simulink model "PID_SingleJoint"  (R2018b)
settings: Solver=FixedStepDiscrete  StartTime=0.0  StopTime=Inf  FixedStep=0.001  RelTol=1e-3  EnableMultiTasking=on
undefined symbols (not defined in the file): DiscIntNeverNeededParam, J1, J2, J3, J4, J5, J6, J7, Motor_Current, Motor_Position, Motor_Velocity, q, qd, Send_GUIdata, Tau
libraries: c280xlib x14, simulink x11, dspsrcs4 x6, idelinklib_common x1
(part 3 of 4)

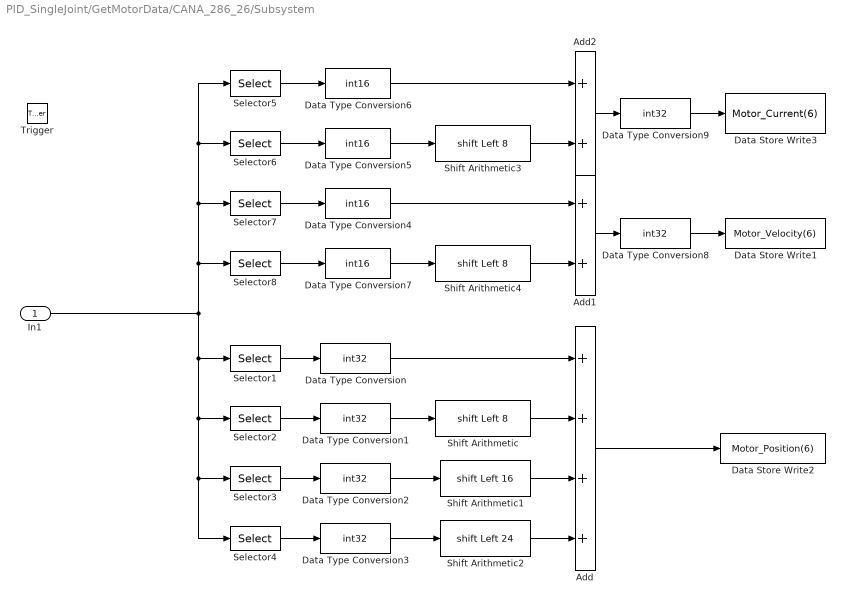
== system PID_SingleJoint/GetMotorData/CANA_286_26/Subsystem ==
  In1 : Inport
  Trigger : TriggerPort  TriggerType=function-call  VariantControl=Variant  PortDimensions=1
  Add : Sum  Inputs=4
  Add1 : Sum  Inputs=2
  Add2 : Sum  Inputs=2
  Data Store Write1 : DataStoreWrite  DataStoreName=Motor_Velocity  DataStoreElements=Motor_Velocity(6)
  Data Store Write2 : DataStoreWrite  DataStoreName=Motor_Position  DataStoreElements=Motor_Position(6)
  Data Store Write3 : DataStoreWrite  DataStoreName=Motor_Current  DataStoreElements=Motor_Current(6)
  Data Type Conversion{,1..3,8..9} (6 alike) : DataTypeConversion  OutDataTypeStr=int32
  Data Type Conversion{4..7} (4 alike) : DataTypeConversion  OutDataTypeStr=int16
  Selector1 : Selector  IndexMode=Zero-based  InputPortWidth=8  IndexOptions=Index vector (dialog)  Indices=4  OutputSizes=1
  Selector2 : Selector  IndexMode=Zero-based  InputPortWidth=8  IndexOptions=Index vector (dialog)  Indices=5  OutputSizes=1
  Selector3 : Selector  IndexMode=Zero-based  InputPortWidth=8  IndexOptions=Index vector (dialog)  Indices=6  OutputSizes=1
  Selector4 : Selector  IndexMode=Zero-based  InputPortWidth=8  IndexOptions=Index vector (dialog)  Indices=7  OutputSizes=1
  Selector5 : Selector  IndexMode=Zero-based  InputPortWidth=8  IndexOptions=Index vector (dialog)  Indices=0  OutputSizes=1
  Selector6 : Selector  IndexMode=Zero-based  InputPortWidth=8  IndexOptions=Index vector (dialog)  Indices=1  OutputSizes=1
  Selector7 : Selector  IndexMode=Zero-based  InputPortWidth=8  IndexOptions=Index vector (dialog)  Indices=2  OutputSizes=1
  Selector8 : Selector  IndexMode=Zero-based  InputPortWidth=8  IndexOptions=Index vector (dialog)  Indices=3  OutputSizes=1
  Shift Arithmetic : ArithShift  BitShiftNumber=8  BitShiftDirection=Left
  Shift Arithmetic1 : ArithShift  BitShiftNumber=16  BitShiftDirection=Left
  Shift Arithmetic2 : ArithShift  BitShiftNumber=24  BitShiftDirection=Left
  Shift Arithmetic3 : ArithShift  BitShiftNumber=8  BitShiftDirection=Left
  Shift Arithmetic4 : ArithShift  BitShiftNumber=8  BitShiftDirection=Left
  wires:
  Selector3/1 -> Data Type Conversion2/1
  Shift Arithmetic/1 -> Add/2
  Shift Arithmetic2/1 -> Add/4
  Data Type Conversion/1 -> Add/1
  Selector1/1 -> Data Type Conversion/1
  Selector4/1 -> Data Type Conversion3/1
  Add/1 -> Data Store Write2/1
  Shift Arithmetic1/1 -> Add/3
  Selector2/1 -> Data Type Conversion1/1
  Selector5/1 -> Data Type Conversion6/1
  Data Type Conversion7/1 -> Shift Arithmetic4/1
  Selector7/1 -> Data Type Conversion4/1
  Selector8/1 -> Data Type Conversion7/1
  Selector6/1 -> Data Type Conversion5/1
  In1/1 -> Selector3/1, Selector4/1, Selector2/1, Selector1/1, Selector5/1, Selector6/1, Selector7/1, Selector8/1
  Add1/1 -> Data Type Conversion8/1
  Data Type Conversion1/1 -> Shift Arithmetic/1
  Data Type Conversion2/1 -> Shift Arithmetic1/1
  Data Type Conversion3/1 -> Shift Arithmetic2/1
  Shift Arithmetic4/1 -> Add1/2
  Data Type Conversion4/1 -> Add1/1
  Data Type Conversion5/1 -> Shift Arithmetic3/1
  Data Type Conversion6/1 -> Add2/1
  Shift Arithmetic3/1 -> Add2/2
  Add2/1 -> Data Type Conversion9/1
  Data Type Conversion8/1 -> Data Store Write1/1
  Data Type Conversion9/1 -> Data Store Write3/1

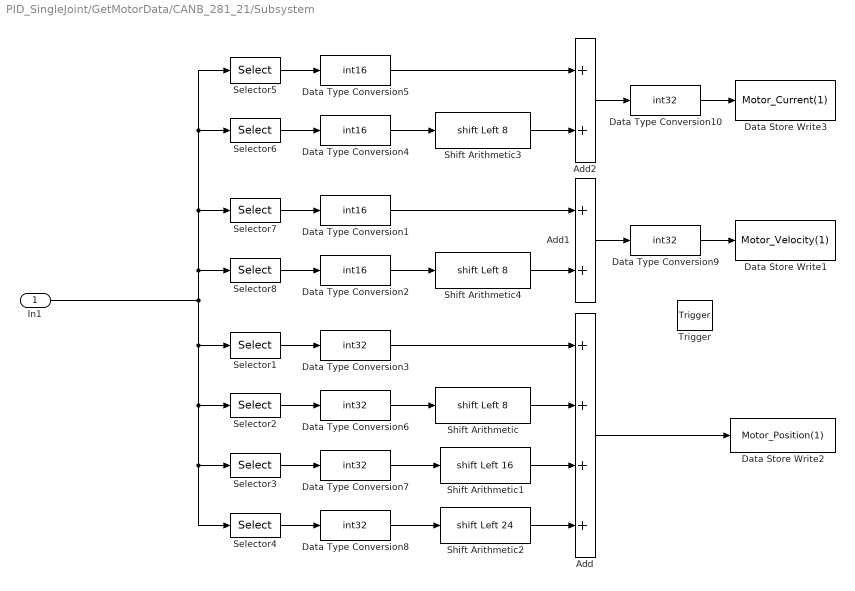
== system PID_SingleJoint/GetMotorData/CANB_281_21/Subsystem ==
  In1 : Inport
  Trigger : TriggerPort  TriggerType=function-call  VariantControl=Variant  PortDimensions=1
  Add : Sum  Inputs=4
  Add1 : Sum  Inputs=2
  Add2 : Sum  Inputs=2
  Data Store Write1 : DataStoreWrite  DataStoreName=Motor_Velocity  DataStoreElements=Motor_Velocity(1)
  Data Store Write2 : DataStoreWrite  DataStoreName=Motor_Position  DataStoreElements=Motor_Position(1)
  Data Store Write3 : DataStoreWrite  DataStoreName=Motor_Current  DataStoreElements=Motor_Current(1)
  Data Type Conversion{1..2,4..5} (4 alike) : DataTypeConversion  OutDataTypeStr=int16
  Data Type Conversion{3,6..10} (6 alike) : DataTypeConversion  OutDataTypeStr=int32
  Selector1 : Selector  IndexMode=Zero-based  InputPortWidth=8  IndexOptions=Index vector (dialog)  Indices=4  OutputSizes=1
  Selector2 : Selector  IndexMode=Zero-based  InputPortWidth=8  IndexOptions=Index vector (dialog)  Indices=5  OutputSizes=1
  Selector3 : Selector  IndexMode=Zero-based  InputPortWidth=8  IndexOptions=Index vector (dialog)  Indices=6  OutputSizes=1
  Selector4 : Selector  IndexMode=Zero-based  InputPortWidth=8  IndexOptions=Index vector (dialog)  Indices=7  OutputSizes=1
  Selector5 : Selector  IndexMode=Zero-based  InputPortWidth=8  IndexOptions=Index vector (dialog)  Indices=0  OutputSizes=1
  Selector6 : Selector  IndexMode=Zero-based  InputPortWidth=8  IndexOptions=Index vector (dialog)  Indices=1  OutputSizes=1
  Selector7 : Selector  IndexMode=Zero-based  InputPortWidth=8  IndexOptions=Index vector (dialog)  Indices=2  OutputSizes=1
  Selector8 : Selector  IndexMode=Zero-based  InputPortWidth=8  IndexOptions=Index vector (dialog)  Indices=3  OutputSizes=1
  Shift Arithmetic : ArithShift  BitShiftNumber=8  BitShiftDirection=Left
  Shift Arithmetic1 : ArithShift  BitShiftNumber=16  BitShiftDirection=Left
  Shift Arithmetic2 : ArithShift  BitShiftNumber=24  BitShiftDirection=Left
  Shift Arithmetic3 : ArithShift  BitShiftNumber=8  BitShiftDirection=Left
  Shift Arithmetic4 : ArithShift  BitShiftNumber=8  BitShiftDirection=Left
  wires:
  Data Type Conversion7/1 -> Shift Arithmetic1/1
  Shift Arithmetic/1 -> Add/2
  Selector2/1 -> Data Type Conversion6/1
  Selector3/1 -> Data Type Conversion7/1
  Shift Arithmetic2/1 -> Add/4
  Data Type Conversion3/1 -> Add/1
  Selector1/1 -> Data Type Conversion3/1
  Data Type Conversion8/1 -> Shift Arithmetic2/1
  Add/1 -> Data Store Write2/1
  Selector4/1 -> Data Type Conversion8/1
  Shift Arithmetic1/1 -> Add/3
  Data Type Conversion6/1 -> Shift Arithmetic/1
  Data Type Conversion2/1 -> Shift Arithmetic4/1
  Shift Arithmetic4/1 -> Add1/2
  Data Type Conversion1/1 -> Add1/1
  Selector7/1 -> Data Type Conversion1/1
  Selector8/1 -> Data Type Conversion2/1
  Selector6/1 -> Data Type Conversion4/1
  In1/1 -> Selector3/1, Selector4/1, Selector2/1, Selector1/1, Selector5/1, Selector6/1, Selector7/1, Selector8/1
  Add1/1 -> Data Type Conversion9/1
  Selector5/1 -> Data Type Conversion5/1
  Data Type Conversion4/1 -> Shift Arithmetic3/1
  Data Type Conversion9/1 -> Data Store Write1/1
  Shift Arithmetic3/1 -> Add2/2
  Data Type Conversion5/1 -> Add2/1
  Add2/1 -> Data Type Conversion10/1
  Data Type Conversion10/1 -> Data Store Write3/1

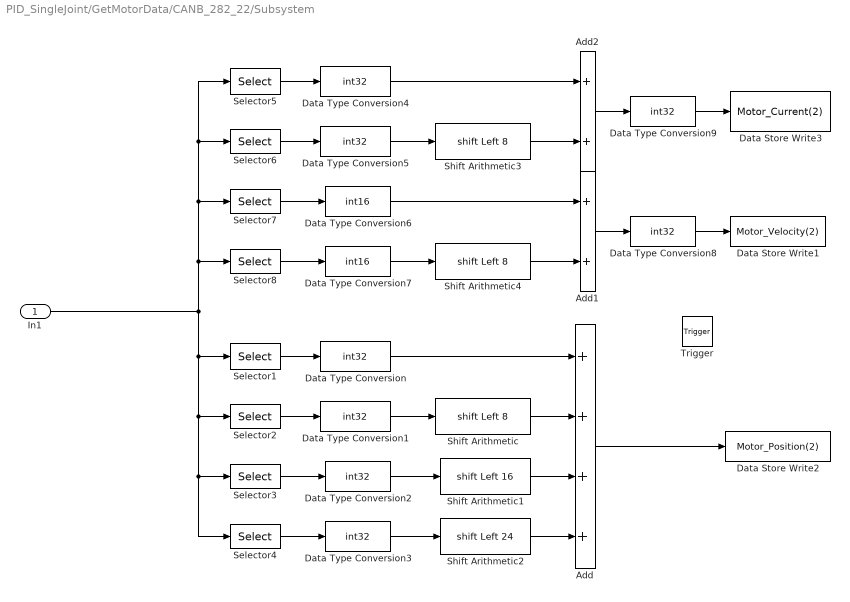
== system PID_SingleJoint/GetMotorData/CANB_282_22/Subsystem ==
  In1 : Inport
  Trigger : TriggerPort  TriggerType=function-call  VariantControl=Variant  PortDimensions=1
  Add : Sum  Inputs=4
  Add1 : Sum  Inputs=2
  Add2 : Sum  Inputs=2
  Data Store Write1 : DataStoreWrite  DataStoreName=Motor_Velocity  DataStoreElements=Motor_Velocity(2)
  Data Store Write2 : DataStoreWrite  DataStoreName=Motor_Position  DataStoreElements=Motor_Position(2)
  Data Store Write3 : DataStoreWrite  DataStoreName=Motor_Current  DataStoreElements=Motor_Current(2)
  Data Type Conversion{,1..5,8..9} (8 alike) : DataTypeConversion  OutDataTypeStr=int32
  Data Type Conversion6 : DataTypeConversion  OutDataTypeStr=int16
  Data Type Conversion7 : DataTypeConversion  OutDataTypeStr=int16
  Selector1 : Selector  IndexMode=Zero-based  InputPortWidth=8  IndexOptions=Index vector (dialog)  Indices=4  OutputSizes=1
  Selector2 : Selector  IndexMode=Zero-based  InputPortWidth=8  IndexOptions=Index vector (dialog)  Indices=5  OutputSizes=1
  Selector3 : Selector  IndexMode=Zero-based  InputPortWidth=8  IndexOptions=Index vector (dialog)  Indices=6  OutputSizes=1
  Selector4 : Selector  IndexMode=Zero-based  InputPortWidth=8  IndexOptions=Index vector (dialog)  Indices=7  OutputSizes=1
  Selector5 : Selector  IndexMode=Zero-based  InputPortWidth=8  IndexOptions=Index vector (dialog)  Indices=0  OutputSizes=1
  Selector6 : Selector  IndexMode=Zero-based  InputPortWidth=8  IndexOptions=Index vector (dialog)  Indices=1  OutputSizes=1
  Selector7 : Selector  IndexMode=Zero-based  InputPortWidth=8  IndexOptions=Index vector (dialog)  Indices=2  OutputSizes=1
  Selector8 : Selector  IndexMode=Zero-based  InputPortWidth=8  IndexOptions=Index vector (dialog)  Indices=3  OutputSizes=1
  Shift Arithmetic : ArithShift  BitShiftNumber=8  BitShiftDirection=Left
  Shift Arithmetic1 : ArithShift  BitShiftNumber=16  BitShiftDirection=Left
  Shift Arithmetic2 : ArithShift  BitShiftNumber=24  BitShiftDirection=Left
  Shift Arithmetic3 : ArithShift  BitShiftNumber=8  BitShiftDirection=Left
  Shift Arithmetic4 : ArithShift  BitShiftNumber=8  BitShiftDirection=Left
  wires:
  Data Type Conversion2/1 -> Shift Arithmetic1/1
  Shift Arithmetic/1 -> Add/2
  Selector2/1 -> Data Type Conversion1/1
  Selector3/1 -> Data Type Conversion2/1
  Shift Arithmetic2/1 -> Add/4
  Data Type Conversion/1 -> Add/1
  Selector1/1 -> Data Type Conversion/1
  Data Type Conversion3/1 -> Shift Arithmetic2/1
  Add/1 -> Data Store Write2/1
  Selector4/1 -> Data Type Conversion3/1
  Shift Arithmetic1/1 -> Add/3
  Data Type Conversion1/1 -> Shift Arithmetic/1
  In1/1 -> Selector3/1, Selector4/1, Selector2/1, Selector1/1, Selector8/1, Selector7/1, Selector6/1, Selector5/1
  Shift Arithmetic4/1 -> Add1/2
  Add1/1 -> Data Type Conversion8/1
  Data Type Conversion5/1 -> Shift Arithmetic3/1
  Selector8/1 -> Data Type Conversion7/1
  Data Type Conversion6/1 -> Add1/1
  Selector6/1 -> Data Type Conversion5/1
  Data Type Conversion7/1 -> Shift Arithmetic4/1
  Selector5/1 -> Data Type Conversion4/1
  Selector7/1 -> Data Type Conversion6/1
  Data Type Conversion8/1 -> Data Store Write1/1
  Shift Arithmetic3/1 -> Add2/2
  Data Type Conversion4/1 -> Add2/1
  Add2/1 -> Data Type Conversion9/1
  Data Type Conversion9/1 -> Data Store Write3/1

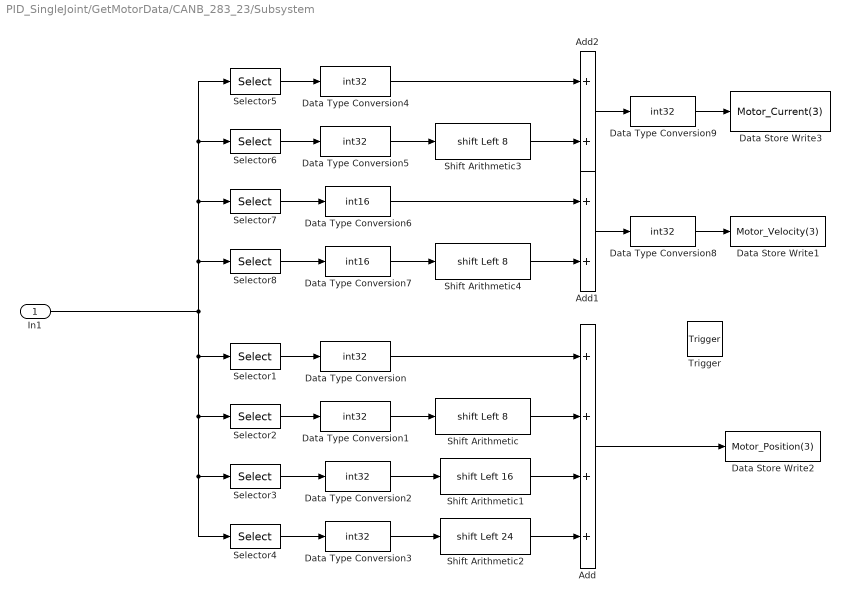
== system PID_SingleJoint/GetMotorData/CANB_283_23/Subsystem ==
  In1 : Inport
  Trigger : TriggerPort  TriggerType=function-call  VariantControl=Variant  PortDimensions=1
  Add : Sum  Inputs=4
  Add1 : Sum  Inputs=2
  Add2 : Sum  Inputs=2
  Data Store Write1 : DataStoreWrite  DataStoreName=Motor_Velocity  DataStoreElements=Motor_Velocity(3)
  Data Store Write2 : DataStoreWrite  DataStoreName=Motor_Position  DataStoreElements=Motor_Position(3)
  Data Store Write3 : DataStoreWrite  DataStoreName=Motor_Current  DataStoreElements=Motor_Current(3)
  Data Type Conversion{,1..5,8..9} (8 alike) : DataTypeConversion  OutDataTypeStr=int32
  Data Type Conversion6 : DataTypeConversion  OutDataTypeStr=int16
  Data Type Conversion7 : DataTypeConversion  OutDataTypeStr=int16
  Selector1 : Selector  IndexMode=Zero-based  InputPortWidth=8  IndexOptions=Index vector (dialog)  Indices=4  OutputSizes=1
  Selector2 : Selector  IndexMode=Zero-based  InputPortWidth=8  IndexOptions=Index vector (dialog)  Indices=5  OutputSizes=1
  Selector3 : Selector  IndexMode=Zero-based  InputPortWidth=8  IndexOptions=Index vector (dialog)  Indices=6  OutputSizes=1
  Selector4 : Selector  IndexMode=Zero-based  InputPortWidth=8  IndexOptions=Index vector (dialog)  Indices=7  OutputSizes=1
  Selector5 : Selector  IndexMode=Zero-based  InputPortWidth=8  IndexOptions=Index vector (dialog)  Indices=0  OutputSizes=1
  Selector6 : Selector  IndexMode=Zero-based  InputPortWidth=8  IndexOptions=Index vector (dialog)  Indices=1  OutputSizes=1
  Selector7 : Selector  IndexMode=Zero-based  InputPortWidth=8  IndexOptions=Index vector (dialog)  Indices=2  OutputSizes=1
  Selector8 : Selector  IndexMode=Zero-based  InputPortWidth=8  IndexOptions=Index vector (dialog)  Indices=3  OutputSizes=1
  Shift Arithmetic : ArithShift  BitShiftNumber=8  BitShiftDirection=Left
  Shift Arithmetic1 : ArithShift  BitShiftNumber=16  BitShiftDirection=Left
  Shift Arithmetic2 : ArithShift  BitShiftNumber=24  BitShiftDirection=Left
  Shift Arithmetic3 : ArithShift  BitShiftNumber=8  BitShiftDirection=Left
  Shift Arithmetic4 : ArithShift  BitShiftNumber=8  BitShiftDirection=Left
  wires:
  Data Type Conversion2/1 -> Shift Arithmetic1/1
  Shift Arithmetic/1 -> Add/2
  Selector2/1 -> Data Type Conversion1/1
  Selector3/1 -> Data Type Conversion2/1
  Shift Arithmetic2/1 -> Add/4
  Data Type Conversion/1 -> Add/1
  Selector1/1 -> Data Type Conversion/1
  Data Type Conversion3/1 -> Shift Arithmetic2/1
  Add/1 -> Data Store Write2/1
  Selector4/1 -> Data Type Conversion3/1
  Shift Arithmetic1/1 -> Add/3
  Data Type Conversion1/1 -> Shift Arithmetic/1
  Selector6/1 -> Data Type Conversion5/1
  Selector5/1 -> Data Type Conversion4/1
  Data Type Conversion7/1 -> Shift Arithmetic4/1
  Data Type Conversion6/1 -> Add1/1
  Selector7/1 -> Data Type Conversion6/1
  Selector8/1 -> Data Type Conversion7/1
  Data Type Conversion5/1 -> Shift Arithmetic3/1
  In1/1 -> Selector3/1, Selector4/1, Selector2/1, Selector1/1, Selector5/1, Selector6/1, Selector7/1, Selector8/1
  Add1/1 -> Data Type Conversion8/1
  Shift Arithmetic4/1 -> Add1/2
  Data Type Conversion8/1 -> Data Store Write1/1
  Shift Arithmetic3/1 -> Add2/2
  Data Type Conversion4/1 -> Add2/1
  Add2/1 -> Data Type Conversion9/1
  Data Type Conversion9/1 -> Data Store Write3/1

== system PID_SingleJoint/接收上位机的数据/Subsystem/Joint1 ==
  Joint1 : Inport
  Action Port : ActionPort  ActionType=case
  Data Store Write2 : DataStoreWrite  DataStoreName=J1
  wires:
  Joint1/1 -> Data Store Write2/1

== system PID_SingleJoint/接收上位机的数据/Subsystem/Joint2 ==
  Joint2 : Inport
  Action Port : ActionPort  ActionType=case
  Data Store Write2 : DataStoreWrite  DataStoreName=J2
  wires:
  Joint2/1 -> Data Store Write2/1

== system PID_SingleJoint/接收上位机的数据/Subsystem/Joint3 ==
  Joint3 : Inport
  Action Port : ActionPort  ActionType=case
  Data Store Write2 : DataStoreWrite  DataStoreName=J3
  wires:
  Joint3/1 -> Data Store Write2/1

== system PID_SingleJoint/接收上位机的数据/Subsystem/Joint4 ==
  Joint4 : Inport
  Action Port : ActionPort  ActionType=case
  Data Store Write2 : DataStoreWrite  DataStoreName=J4
  wires:
  Joint4/1 -> Data Store Write2/1

== system PID_SingleJoint/接收上位机的数据/Subsystem/Joint5 ==
  Joint5 : Inport
  Action Port : ActionPort  ActionType=case
  Data Store Write2 : DataStoreWrite  DataStoreName=J5
  wires:
  Joint5/1 -> Data Store Write2/1

== system PID_SingleJoint/接收上位机的数据/Subsystem/Joint6 ==
  Joint6 : Inport
  Action Port : ActionPort  ActionType=case
  Data Store Write2 : DataStoreWrite  DataStoreName=J6
  wires:
  Joint6/1 -> Data Store Write2/1

== system PID_SingleJoint/接收上位机的数据/Subsystem/Joint7 ==
  Joint7 : Inport
  Action Port : ActionPort  ActionType=case
  Data Store Write2 : DataStoreWrite  DataStoreName=J7
  wires:
  Joint7/1 -> Data Store Write2/1

== system PID_SingleJoint/接收上位机的数据/获取用户命令/消息校验 ==
  数据 : Inport
  Add : Sum  Inputs=8
  Constant : Constant  Value=[0 0 0 0 0 0 0 0 0]  OutDataTypeStr=uint16
  Data Type Conversion : DataTypeConversion  OutDataTypeStr=uint16
  Demux : Demux  Outputs=9
  Relational Operator : RelationalOperator  Operator===  OutDataTypeStr=boolean  RndMeth=Simplest
  Switch : Switch  Criteria=u2 > Threshold
  消息 : Outport
  使能 : Outport  Port=2
  wires:
  数据/1 -> Switch/1, Demux/1
  Demux/1 -> Add/1
  Demux/2 -> Add/2
  Demux/3 -> Add/3
  Demux/4 -> Add/4
  Demux/5 -> Add/5
  Demux/6 -> Add/6
  Demux/7 -> Add/7
  Demux/8 -> Add/8
  Add/1 -> Data Type Conversion/1
  Data Type Conversion/1 -> Relational Operator/1
  Demux/9 -> Relational Operator/2
  Switch/1 -> 消息/1
  Constant/1 -> Switch/3
  Relational Operator/1 -> Switch/2, 使能/1

== system PID_SingleJoint/DynamicsController/DriveMotor/BottomDriver/Joint1 ==
  In6 : Inport
  eCANB_301_7 : c280xlib/eCAN Transmit  chipFamily=C280x  useModule=eCAN_B  mailboxNo=7  messageID=hex2dec('301')  messageType=Standard (11-bit identifier)  enableBlockingMode=off  postInterrupt=off  interruptLine=0
      settings: SourceProductName=Embedded Coder Support Package for Texas Instruments C2000 Processors  SourceProductBaseCode=TIC2000
  wires:
  In6/1 -> eCANB_301_7/1

== system PID_SingleJoint/DynamicsController/DriveMotor/BottomDriver/Joint2 ==
  In1 : Inport
  eCANB _302_8 : c280xlib/eCAN Transmit  chipFamily=C280x  useModule=eCAN_B  mailboxNo=8  messageID=hex2dec('302')  messageType=Standard (11-bit identifier)  enableBlockingMode=off  postInterrupt=off  interruptLine=0
      settings: SourceProductName=Embedded Coder Support Package for Texas Instruments C2000 Processors  SourceProductBaseCode=TIC2000
  wires:
  In1/1 -> eCANB _302_8/1

== system PID_SingleJoint/DynamicsController/DriveMotor/BottomDriver/Joint3 ==
  In1 : Inport
  eCANB _303_9 : c280xlib/eCAN Transmit  chipFamily=C280x  useModule=eCAN_B  mailboxNo=9  messageID=hex2dec('303')  messageType=Standard (11-bit identifier)  enableBlockingMode=off  postInterrupt=off  interruptLine=0
      settings: SourceProductName=Embedded Coder Support Package for Texas Instruments C2000 Processors  SourceProductBaseCode=TIC2000
  wires:
  In1/1 -> eCANB _303_9/1

== system PID_SingleJoint/DynamicsController/DriveMotor/BottomDriver/Joint4 ==
  In1 : Inport
  eCANA_304_10 : c280xlib/eCAN Transmit  chipFamily=C280x  useModule=eCAN_A  mailboxNo=10  messageID=hex2dec('304')  messageType=Standard (11-bit identifier)  enableBlockingMode=off  postInterrupt=off  interruptLine=0
      settings: SourceProductName=Embedded Coder Support Package for Texas Instruments C2000 Processors  SourceProductBaseCode=TIC2000
  wires:
  In1/1 -> eCANA_304_10/1

== system PID_SingleJoint/DynamicsController/DriveMotor/BottomDriver/Joint5 ==
  In1 : Inport
  eCANA_305_11 : c280xlib/eCAN Transmit  chipFamily=C280x  useModule=eCAN_A  mailboxNo=11  messageID=hex2dec('305')  messageType=Standard (11-bit identifier)  enableBlockingMode=off  postInterrupt=off  interruptLine=0
      settings: SourceProductName=Embedded Coder Support Package for Texas Instruments C2000 Processors  SourceProductBaseCode=TIC2000
  wires:
  In1/1 -> eCANA_305_11/1

== system PID_SingleJoint/DynamicsController/DriveMotor/BottomDriver/Joint6 ==
  In1 : Inport
  eCANA_306_12 : c280xlib/eCAN Transmit  chipFamily=C280x  useModule=eCAN_A  mailboxNo=12  messageID=hex2dec('306')  messageType=Standard (11-bit identifier)  enableBlockingMode=off  postInterrupt=off  interruptLine=0
      settings: SourceProductName=Embedded Coder Support Package for Texas Instruments C2000 Processors  SourceProductBaseCode=TIC2000
  wires:
  In1/1 -> eCANA_306_12/1

== system PID_SingleJoint/DynamicsController/DriveMotor/驱动器指令/Chart2/BG ==
  f : TriggerPort  TriggerType=function-call  VariantControl=(inherit)
      settings: CopyFcn=Stateflow.SLINSF.SimulinkMan.removeBlockPreDeleteFcn  PreDeleteFcn=Stateflow.SLINSF.SimulinkMan.unsafePredeleteFcn
  Constant6 : Constant  OutDataTypeStr=uint8
  Data Store Write : DataStoreWrite  DataStoreName=TXD
  J1_BG : Subsystem  TreatAsAtomicUnit=on
  J2_BG : Subsystem  TreatAsAtomicUnit=on
  J3_BG : Subsystem  TreatAsAtomicUnit=on
  J4_BG : Subsystem  TreatAsAtomicUnit=on
  J5_BG : Subsystem  TreatAsAtomicUnit=on
  J6_BG : Subsystem  TreatAsAtomicUnit=on
  Mux1 : Mux  Inputs=3
  Mux2 : Mux  Inputs=3
  Mux3 : Mux  Inputs=2
  Reshape1 : Reshape  OutputDimensionality=Customize  OutputDimensions=[1,24]
  Reshape2 : Reshape  OutputDimensionality=Customize  OutputDimensions=[1,24]
  Reshape6 : Reshape  OutputDimensionality=Customize  OutputDimensions=[1,48]
  MSG : Outport
  wires:
  Constant6/1 -> Data Store Write/1
  J1_BG/1(MSG) -> Mux1/1
  J2_BG/1(MSG) -> Mux1/2
  J3_BG/1(MSG) -> Mux1/3
  J4_BG/1(MSG) -> Mux2/1
  J5_BG/1(MSG) -> Mux2/2
  J6_BG/1(MSG) -> Mux2/3
  Mux1/1 -> Reshape1/1
  Mux2/1 -> Reshape2/1
  Mux3/1 -> Reshape6/1
  Reshape6/1 -> MSG/1
  Reshape1/1 -> Mux3/1
  Reshape2/1 -> Mux3/2

== system PID_SingleJoint/DynamicsController/DriveMotor/驱动器指令/Chart2/TF ==
  Current : Inport  OutDataTypeStr=uint16  PortDimensions=[1 6]
  f : TriggerPort  TriggerType=function-call  VariantControl=(inherit)
      settings: CopyFcn=Stateflow.SLINSF.SimulinkMan.removeBlockPreDeleteFcn  PreDeleteFcn=Stateflow.SLINSF.SimulinkMan.unsafePredeleteFcn
  Constant2 : Constant  OutDataTypeStr=uint8
  Data Store Write : DataStoreWrite  DataStoreName=TXD
  Demux : Demux  Outputs=6
  J1_TF : Subsystem  TreatAsAtomicUnit=on
  J2_TF : Subsystem  TreatAsAtomicUnit=on
  J3_TF : Subsystem  TreatAsAtomicUnit=on
  J4_TF : Subsystem  TreatAsAtomicUnit=on
  J5_TF : Subsystem  TreatAsAtomicUnit=on
  J6_TF : Subsystem  TreatAsAtomicUnit=on
  Mux3 : Mux  Inputs=6
  Reshape{,1..5} (6 alike) : Reshape  OutputDimensionality=Customize  OutputDimensions=[1,8]
  Reshape6 : Reshape  OutputDimensionality=Customize  OutputDimensions=[1,48]
  MSG : Outport
  wires:
  Constant2/1 -> Data Store Write/1
  J1_TF/1(MSG) -> Reshape/1
  J2_TF/1(MSG) -> Reshape1/1
  J3_TF/1(MSG) -> Reshape2/1
  J4_TF/1(MSG) -> Reshape3/1
  J5_TF/1(MSG) -> Reshape4/1
  J6_TF/1(MSG) -> Reshape5/1
  Mux3/1 -> Reshape6/1
  Demux/1 -> J1_TF/1(Current)
  Demux/2 -> J2_TF/1(Current)
  Demux/3 -> J3_TF/1(Current)
  Demux/4 -> J4_TF/1(Current)
  Demux/5 -> J5_TF/1(Current)
  Demux/6 -> J6_TF/1(Current)
  Current/1 -> Demux/1
  Reshape/1 -> Mux3/1
  Reshape1/1 -> Mux3/2
  Reshape2/1 -> Mux3/3
  Reshape3/1 -> Mux3/4
  Reshape4/1 -> Mux3/5
  Reshape5/1 -> Mux3/6
  Reshape6/1 -> MSG/1

== system PID_SingleJoint/DynamicsController/DriveMotor/驱动器指令/Chart2/UM1 ==
  f : TriggerPort  TriggerType=function-call  VariantControl=(inherit)
      settings: CopyFcn=Stateflow.SLINSF.SimulinkMan.removeBlockPreDeleteFcn  PreDeleteFcn=Stateflow.SLINSF.SimulinkMan.unsafePredeleteFcn
  Constant : Constant  OutDataTypeStr=uint8
  Data Store Write : DataStoreWrite  DataStoreName=TXD
  J1_UM1 : Subsystem  TreatAsAtomicUnit=on
      settings: RTWSystemCode=Nonreusable function
  J2_UM1 : Subsystem  TreatAsAtomicUnit=on
      settings: RTWSystemCode=Nonreusable function
  J3_UM1 : Subsystem  TreatAsAtomicUnit=on
      settings: RTWSystemCode=Nonreusable function
  J4_UM1 : Subsystem  TreatAsAtomicUnit=on
      settings: RTWSystemCode=Nonreusable function
  J5_UM1 : Subsystem  TreatAsAtomicUnit=on
      settings: RTWSystemCode=Nonreusable function
  J6_UM1 : Subsystem  TreatAsAtomicUnit=on
      settings: RTWSystemCode=Nonreusable function
  Mux : Mux  Inputs=3
  Mux1 : Mux  Inputs=3
  Mux2 : Mux  Inputs=2
  Reshape1 : Reshape  OutputDimensionality=Customize  OutputDimensions=[1,48]
  Reshape2 : Reshape  OutputDimensionality=Customize  OutputDimensions=[1,24]
  Reshape3 : Reshape  OutputDimensionality=Customize  OutputDimensions=[1,24]
  MSG : Outport
  wires:
  Constant/1 -> Data Store Write/1
  J4_UM1/1(MSG) -> Mux/1
  J6_UM1/1(MSG) -> Mux/3
  J5_UM1/1(MSG) -> Mux/2
  J2_UM1/1(MSG) -> Mux1/2
  J3_UM1/1(MSG) -> Mux1/3
  J1_UM1/1(MSG) -> Mux1/1
  Mux1/1 -> Reshape2/1
  Mux/1 -> Reshape3/1
  Mux2/1 -> Reshape1/1
  Reshape1/1 -> MSG/1
  Reshape2/1 -> Mux2/1
  Reshape3/1 -> Mux2/2

== system PID_SingleJoint/DynamicsController/DriveMotor/驱动器指令/Chart2/check ==
  write : Inport  OutDataTypeStr=uint16  PortDimensions=1
  f : TriggerPort  TriggerType=function-call  VariantControl=(inherit)
      settings: CopyFcn=Stateflow.SLINSF.SimulinkMan.removeBlockPreDeleteFcn  PreDeleteFcn=Stateflow.SLINSF.SimulinkMan.unsafePredeleteFcn
  Constant : Constant  OutDataTypeStr=uint16
  Constant1 : Constant  Value=0  OutDataTypeStr=uint16
  Data Type Conversion : DataTypeConversion  OutDataTypeStr=uint16
  Switch : Switch  Criteria=u2 > Threshold  OutDataTypeStr=uint16
  bx : Outport  OutDataTypeStr=uint16  PortDimensions=1
  wires:
  Switch/1 -> Data Type Conversion/1
  Constant1/1 -> Switch/3
  Constant/1 -> Switch/1
  write/1 -> Switch/2
  Data Type Conversion/1 -> bx/1

== system PID_SingleJoint/DynamicsController/DriveMotor/驱动器指令/Chart2/start_arm ==
  StartRobot : Inport  OutDataTypeStr=uint16  PortDimensions=1
  f : TriggerPort  TriggerType=function-call  VariantControl=(inherit)
      settings: CopyFcn=Stateflow.SLINSF.SimulinkMan.removeBlockPreDeleteFcn  PreDeleteFcn=Stateflow.SLINSF.SimulinkMan.unsafePredeleteFcn
  Constant : Constant  OutDataTypeStr=uint16
  StartRobotSubsystem : Subsystem
      settings: RTWSystemCode=Nonreusable function
  start : Outport  OutDataTypeStr=uint16  PortDimensions=1
  wires:
  StartRobot/1 -> StartRobotSubsystem/Enable
  StartRobotSubsystem/1(Out1) -> start/1
  Constant/1 -> StartRobotSubsystem/1(In1)

== system PID_SingleJoint/DynamicsController/GetAngleVelocity/GetAngle1/Joint1 ==
  note: 内转子位置的脉冲值
  Action Port : ActionPort
  Data Store Read5 : DataStoreRead  DataStoreName=Motor_Position  DataStoreElements=Motor_Position(1)
  Joint1 : Outport
  wires:
  Data Store Read5/1 -> Joint1/1

== system PID_SingleJoint/DynamicsController/GetAngleVelocity/GetAngle1/Joint2 ==
  Action Port : ActionPort
  Data Store Read5 : DataStoreRead  DataStoreName=Motor_Position  DataStoreElements=Motor_Position(2)
  Joint2 : Outport
  wires:
  Data Store Read5/1 -> Joint2/1

== system PID_SingleJoint/DynamicsController/GetAngleVelocity/GetAngle1/Joint3 ==
  Action Port : ActionPort
  Data Store Read5 : DataStoreRead  DataStoreName=Motor_Position  DataStoreElements=Motor_Position(3)
  Joint3 : Outport
  wires:
  Data Store Read5/1 -> Joint3/1

== system PID_SingleJoint/DynamicsController/GetAngleVelocity/GetAngle1/Joint4 ==
  Action Port : ActionPort
  Data Store Read5 : DataStoreRead  DataStoreName=Motor_Position  DataStoreElements=Motor_Position(4)
  Joint4 : Outport
  wires:
  Data Store Read5/1 -> Joint4/1

== system PID_SingleJoint/DynamicsController/GetAngleVelocity/GetAngle1/Joint5 ==
  Action Port : ActionPort
  Data Store Read5 : DataStoreRead  DataStoreName=Motor_Position  DataStoreElements=Motor_Position(5)
  Joint5 : Outport
  wires:
  Data Store Read5/1 -> Joint5/1

== system PID_SingleJoint/DynamicsController/GetAngleVelocity/GetAngle1/Joint6 ==
  Action Port : ActionPort
  Data Store Read5 : DataStoreRead  DataStoreName=Motor_Position  DataStoreElements=Motor_Position(6)
  Joint6 : Outport
  wires:
  Data Store Read5/1 -> Joint6/1

== system PID_SingleJoint/DynamicsController/GetAngleVelocity/GetAngle2/Joint1 ==
  note: 内转子位置的脉冲值
  Action Port : ActionPort
  Data Store Read5 : DataStoreRead  DataStoreName=Motor_Position  DataStoreElements=Motor_Position(1)
  Joint1 : Outport
  wires:
  Data Store Read5/1 -> Joint1/1

== system PID_SingleJoint/DynamicsController/GetAngleVelocity/GetAngle2/Joint2 ==
  Action Port : ActionPort
  Data Store Read5 : DataStoreRead  DataStoreName=Motor_Position  DataStoreElements=Motor_Position(2)
  Joint2 : Outport
  wires:
  Data Store Read5/1 -> Joint2/1

== system PID_SingleJoint/DynamicsController/GetAngleVelocity/GetAngle2/Joint3 ==
  Action Port : ActionPort
  Data Store Read5 : DataStoreRead  DataStoreName=Motor_Position  DataStoreElements=Motor_Position(3)
  Joint3 : Outport
  wires:
  Data Store Read5/1 -> Joint3/1

== system PID_SingleJoint/DynamicsController/GetAngleVelocity/GetAngle2/Joint4 ==
  Action Port : ActionPort
  Data Store Read5 : DataStoreRead  DataStoreName=Motor_Position  DataStoreElements=Motor_Position(4)
  Joint4 : Outport
  wires:
  Data Store Read5/1 -> Joint4/1

== system PID_SingleJoint/DynamicsController/GetAngleVelocity/GetAngle2/Joint5 ==
  Action Port : ActionPort
  Data Store Read5 : DataStoreRead  DataStoreName=Motor_Position  DataStoreElements=Motor_Position(5)
  Joint5 : Outport
  wires:
  Data Store Read5/1 -> Joint5/1

== system PID_SingleJoint/DynamicsController/GetAngleVelocity/GetAngle2/Joint6 ==
  Action Port : ActionPort
  Data Store Read5 : DataStoreRead  DataStoreName=Motor_Position  DataStoreElements=Motor_Position(6)
  Joint6 : Outport
  wires:
  Data Store Read5/1 -> Joint6/1

== system PID_SingleJoint/DynamicsController/GetAngleVelocity/GetAngle3/Joint1 ==
  note: 内转子位置的脉冲值
  Action Port : ActionPort
  Data Store Read5 : DataStoreRead  DataStoreName=Motor_Position  DataStoreElements=Motor_Position(1)
  Joint1 : Outport
  wires:
  Data Store Read5/1 -> Joint1/1

== system PID_SingleJoint/DynamicsController/GetAngleVelocity/GetAngle3/Joint2 ==
  Action Port : ActionPort
  Data Store Read5 : DataStoreRead  DataStoreName=Motor_Position  DataStoreElements=Motor_Position(2)
  Joint2 : Outport
  wires:
  Data Store Read5/1 -> Joint2/1

== system PID_SingleJoint/DynamicsController/GetAngleVelocity/GetAngle3/Joint3 ==
  Action Port : ActionPort
  Data Store Read5 : DataStoreRead  DataStoreName=Motor_Position  DataStoreElements=Motor_Position(3)
  Joint3 : Outport
  wires:
  Data Store Read5/1 -> Joint3/1

== system PID_SingleJoint/DynamicsController/GetAngleVelocity/GetAngle3/Joint4 ==
  Action Port : ActionPort
  Data Store Read5 : DataStoreRead  DataStoreName=Motor_Position  DataStoreElements=Motor_Position(4)
  Joint4 : Outport
  wires:
  Data Store Read5/1 -> Joint4/1

== system PID_SingleJoint/DynamicsController/GetAngleVelocity/GetAngle3/Joint5 ==
  Action Port : ActionPort
  Data Store Read5 : DataStoreRead  DataStoreName=Motor_Position  DataStoreElements=Motor_Position(5)
  Joint5 : Outport
  wires:
  Data Store Read5/1 -> Joint5/1

== system PID_SingleJoint/DynamicsController/GetAngleVelocity/GetAngle3/Joint6 ==
  Action Port : ActionPort
  Data Store Read5 : DataStoreRead  DataStoreName=Motor_Position  DataStoreElements=Motor_Position(6)
  Joint6 : Outport
  wires:
  Data Store Read5/1 -> Joint6/1

== system PID_SingleJoint/DynamicsController/GetAngleVelocity/GetAngle4/Joint1 ==
  note: 内转子位置的脉冲值
  Action Port : ActionPort
  Data Store Read5 : DataStoreRead  DataStoreName=Motor_Position  DataStoreElements=Motor_Position(1)
  Joint1 : Outport
  wires:
  Data Store Read5/1 -> Joint1/1

== system PID_SingleJoint/DynamicsController/GetAngleVelocity/GetAngle4/Joint2 ==
  Action Port : ActionPort
  Data Store Read5 : DataStoreRead  DataStoreName=Motor_Position  DataStoreElements=Motor_Position(2)
  Joint2 : Outport
  wires:
  Data Store Read5/1 -> Joint2/1

== system PID_SingleJoint/DynamicsController/GetAngleVelocity/GetAngle4/Joint3 ==
  Action Port : ActionPort
  Data Store Read5 : DataStoreRead  DataStoreName=Motor_Position  DataStoreElements=Motor_Position(3)
  Joint3 : Outport
  wires:
  Data Store Read5/1 -> Joint3/1

== system PID_SingleJoint/DynamicsController/GetAngleVelocity/GetAngle4/Joint4 ==
  Action Port : ActionPort
  Data Store Read5 : DataStoreRead  DataStoreName=Motor_Position  DataStoreElements=Motor_Position(4)
  Joint4 : Outport
  wires:
  Data Store Read5/1 -> Joint4/1

== system PID_SingleJoint/DynamicsController/GetAngleVelocity/GetAngle4/Joint5 ==
  Action Port : ActionPort
  Data Store Read5 : DataStoreRead  DataStoreName=Motor_Position  DataStoreElements=Motor_Position(5)
  Joint5 : Outport
  wires:
  Data Store Read5/1 -> Joint5/1

== system PID_SingleJoint/DynamicsController/GetAngleVelocity/GetAngle4/Joint6 ==
  Action Port : ActionPort
  Data Store Read5 : DataStoreRead  DataStoreName=Motor_Position  DataStoreElements=Motor_Position(6)
  Joint6 : Outport
  wires:
  Data Store Read5/1 -> Joint6/1

== system PID_SingleJoint/DynamicsController/GetAngleVelocity/GetAngle5/Joint1 ==
  note: 内转子位置的脉冲值
  Action Port : ActionPort
  Data Store Read5 : DataStoreRead  DataStoreName=Motor_Position  DataStoreElements=Motor_Position(1)
  Joint1 : Outport
  wires:
  Data Store Read5/1 -> Joint1/1

== system PID_SingleJoint/DynamicsController/GetAngleVelocity/GetAngle5/Joint2 ==
  Action Port : ActionPort
  Data Store Read5 : DataStoreRead  DataStoreName=Motor_Position  DataStoreElements=Motor_Position(2)
  Joint2 : Outport
  wires:
  Data Store Read5/1 -> Joint2/1

== system PID_SingleJoint/DynamicsController/GetAngleVelocity/GetAngle5/Joint3 ==
  Action Port : ActionPort
  Data Store Read5 : DataStoreRead  DataStoreName=Motor_Position  DataStoreElements=Motor_Position(3)
  Joint3 : Outport
  wires:
  Data Store Read5/1 -> Joint3/1

== system PID_SingleJoint/DynamicsController/GetAngleVelocity/GetAngle5/Joint4 ==
  Action Port : ActionPort
  Data Store Read5 : DataStoreRead  DataStoreName=Motor_Position  DataStoreElements=Motor_Position(4)
  Joint4 : Outport
  wires:
  Data Store Read5/1 -> Joint4/1

== system PID_SingleJoint/DynamicsController/GetAngleVelocity/GetAngle5/Joint5 ==
  Action Port : ActionPort
  Data Store Read5 : DataStoreRead  DataStoreName=Motor_Position  DataStoreElements=Motor_Position(5)
  Joint5 : Outport
  wires:
  Data Store Read5/1 -> Joint5/1

== system PID_SingleJoint/DynamicsController/GetAngleVelocity/GetAngle5/Joint6 ==
  Action Port : ActionPort
  Data Store Read5 : DataStoreRead  DataStoreName=Motor_Position  DataStoreElements=Motor_Position(6)
  Joint6 : Outport
  wires:
  Data Store Read5/1 -> Joint6/1

== system PID_SingleJoint/DynamicsController/GetAngleVelocity/GetAngle6/Joint1 ==
  note: 内转子位置的脉冲值
  Action Port : ActionPort
  Data Store Read5 : DataStoreRead  DataStoreName=Motor_Position  DataStoreElements=Motor_Position(1)
  Joint1 : Outport
  wires:
  Data Store Read5/1 -> Joint1/1

== system PID_SingleJoint/DynamicsController/GetAngleVelocity/GetAngle6/Joint2 ==
  Action Port : ActionPort
  Data Store Read5 : DataStoreRead  DataStoreName=Motor_Position  DataStoreElements=Motor_Position(2)
  Joint2 : Outport
  wires:
  Data Store Read5/1 -> Joint2/1

== system PID_SingleJoint/DynamicsController/GetAngleVelocity/GetAngle6/Joint3 ==
  Action Port : ActionPort
  Data Store Read5 : DataStoreRead  DataStoreName=Motor_Position  DataStoreElements=Motor_Position(3)
  Joint3 : Outport
  wires:
  Data Store Read5/1 -> Joint3/1

== system PID_SingleJoint/DynamicsController/GetAngleVelocity/GetAngle6/Joint4 ==
  Action Port : ActionPort
  Data Store Read5 : DataStoreRead  DataStoreName=Motor_Position  DataStoreElements=Motor_Position(4)
  Joint4 : Outport
  wires:
  Data Store Read5/1 -> Joint4/1

== system PID_SingleJoint/DynamicsController/GetAngleVelocity/GetAngle6/Joint5 ==
  Action Port : ActionPort
  Data Store Read5 : DataStoreRead  DataStoreName=Motor_Position  DataStoreElements=Motor_Position(5)
  Joint5 : Outport
  wires:
  Data Store Read5/1 -> Joint5/1

== system PID_SingleJoint/DynamicsController/GetAngleVelocity/GetAngle6/Joint6 ==
  Action Port : ActionPort
  Data Store Read5 : DataStoreRead  DataStoreName=Motor_Position  DataStoreElements=Motor_Position(6)
  Joint6 : Outport
  wires:
  Data Store Read5/1 -> Joint6/1

== system PID_SingleJoint/DynamicsController/GetAngleVelocity/GetAngleSpeed/Joint1 ==
  note: 内转子速度
      | 的脉冲值
  Action Port : ActionPort
  Data Store Read1 : DataStoreRead  DataStoreName=Motor_Velocity  DataStoreElements=Motor_Velocity(1)
  Joint1_Velocity : Outport
  wires:
  Data Store Read1/1 -> Joint1_Velocity/1

== system PID_SingleJoint/DynamicsController/GetAngleVelocity/GetAngleSpeed/Joint2 ==
  note: 内转子速度
      | 的脉冲值
  Action Port : ActionPort
  Data Store Read1 : DataStoreRead  DataStoreName=Motor_Velocity  DataStoreElements=Motor_Velocity(2)
  Joint2_Velocity : Outport
  wires:
  Data Store Read1/1 -> Joint2_Velocity/1

== system PID_SingleJoint/DynamicsController/GetAngleVelocity/GetAngleSpeed/Joint3 ==
  note: 内转子速度
      | 的脉冲值
  Action Port : ActionPort
  Data Store Read1 : DataStoreRead  DataStoreName=Motor_Velocity  DataStoreElements=Motor_Velocity(3)
  Joint3_Velocity : Outport
  wires:
  Data Store Read1/1 -> Joint3_Velocity/1

== system PID_SingleJoint/DynamicsController/GetAngleVelocity/GetAngleSpeed/Joint4 ==
  note: 内转子速度
      | 的脉冲值
  Action Port : ActionPort
  Data Store Read1 : DataStoreRead  DataStoreName=Motor_Velocity  DataStoreElements=Motor_Velocity(4)
  Joint4_Velocity : Outport
  wires:
  Data Store Read1/1 -> Joint4_Velocity/1

== system PID_SingleJoint/DynamicsController/GetAngleVelocity/GetAngleSpeed/Joint5 ==
  note: 内转子速度
      | 的脉冲值
  Action Port : ActionPort
  Data Store Read1 : DataStoreRead  DataStoreName=Motor_Velocity  DataStoreElements=Motor_Velocity(5)
  Joint5_Velocity : Outport
  wires:
  Data Store Read1/1 -> Joint5_Velocity/1

== system PID_SingleJoint/DynamicsController/GetAngleVelocity/GetAngleSpeed/Joint6 ==
  note: 内转子速度
      | 的脉冲值
  Action Port : ActionPort
  Data Store Read1 : DataStoreRead  DataStoreName=Motor_Velocity  DataStoreElements=Motor_Velocity(6)
  Joint6_Velocity : Outport
  wires:
  Data Store Read1/1 -> Joint6_Velocity/1

== system PID_SingleJoint/DynamicsController/GetAngleVelocity/GetAngleSpeed1/Joint1 ==
  note: 内转子速度
      | 的脉冲值
  Action Port : ActionPort
  Data Store Read1 : DataStoreRead  DataStoreName=Motor_Velocity  DataStoreElements=Motor_Velocity(1)
  Joint1_Velocity : Outport
  wires:
  Data Store Read1/1 -> Joint1_Velocity/1

== system PID_SingleJoint/DynamicsController/GetAngleVelocity/GetAngleSpeed1/Joint2 ==
  note: 内转子速度
      | 的脉冲值
  Action Port : ActionPort
  Data Store Read1 : DataStoreRead  DataStoreName=Motor_Velocity  DataStoreElements=Motor_Velocity(2)
  Joint2_Velocity : Outport
  wires:
  Data Store Read1/1 -> Joint2_Velocity/1

== system PID_SingleJoint/DynamicsController/GetAngleVelocity/GetAngleSpeed1/Joint3 ==
  note: 内转子速度
      | 的脉冲值
  Action Port : ActionPort
  Data Store Read1 : DataStoreRead  DataStoreName=Motor_Velocity  DataStoreElements=Motor_Velocity(3)
  Joint3_Velocity : Outport
  wires:
  Data Store Read1/1 -> Joint3_Velocity/1

== system PID_SingleJoint/DynamicsController/GetAngleVelocity/GetAngleSpeed1/Joint4 ==
  note: 内转子速度
      | 的脉冲值
  Action Port : ActionPort
  Data Store Read1 : DataStoreRead  DataStoreName=Motor_Velocity  DataStoreElements=Motor_Velocity(4)
  Joint4_Velocity : Outport
  wires:
  Data Store Read1/1 -> Joint4_Velocity/1

== system PID_SingleJoint/DynamicsController/GetAngleVelocity/GetAngleSpeed1/Joint5 ==
  note: 内转子速度
      | 的脉冲值
  Action Port : ActionPort
  Data Store Read1 : DataStoreRead  DataStoreName=Motor_Velocity  DataStoreElements=Motor_Velocity(5)
  Joint5_Velocity : Outport
  wires:
  Data Store Read1/1 -> Joint5_Velocity/1

== system PID_SingleJoint/DynamicsController/GetAngleVelocity/GetAngleSpeed1/Joint6 ==
  note: 内转子速度
      | 的脉冲值
  Action Port : ActionPort
  Data Store Read1 : DataStoreRead  DataStoreName=Motor_Velocity  DataStoreElements=Motor_Velocity(6)
  Joint6_Velocity : Outport
  wires:
  Data Store Read1/1 -> Joint6_Velocity/1

== system PID_SingleJoint/DynamicsController/GetAngleVelocity/GetAngleSpeed2/Joint1 ==
  note: 内转子速度
      | 的脉冲值
  Action Port : ActionPort
  Data Store Read1 : DataStoreRead  DataStoreName=Motor_Velocity  DataStoreElements=Motor_Velocity(1)
  Joint1_Velocity : Outport
  wires:
  Data Store Read1/1 -> Joint1_Velocity/1

== system PID_SingleJoint/DynamicsController/GetAngleVelocity/GetAngleSpeed2/Joint2 ==
  note: 内转子速度
      | 的脉冲值
  Action Port : ActionPort
  Data Store Read1 : DataStoreRead  DataStoreName=Motor_Velocity  DataStoreElements=Motor_Velocity(2)
  Joint2_Velocity : Outport
  wires:
  Data Store Read1/1 -> Joint2_Velocity/1

== system PID_SingleJoint/DynamicsController/GetAngleVelocity/GetAngleSpeed2/Joint3 ==
  note: 内转子速度
      | 的脉冲值
  Action Port : ActionPort
  Data Store Read1 : DataStoreRead  DataStoreName=Motor_Velocity  DataStoreElements=Motor_Velocity(3)
  Joint3_Velocity : Outport
  wires:
  Data Store Read1/1 -> Joint3_Velocity/1

== system PID_SingleJoint/DynamicsController/GetAngleVelocity/GetAngleSpeed2/Joint4 ==
  note: 内转子速度
      | 的脉冲值
  Action Port : ActionPort
  Data Store Read1 : DataStoreRead  DataStoreName=Motor_Velocity  DataStoreElements=Motor_Velocity(4)
  Joint4_Velocity : Outport
  wires:
  Data Store Read1/1 -> Joint4_Velocity/1

== system PID_SingleJoint/DynamicsController/GetAngleVelocity/GetAngleSpeed2/Joint5 ==
  note: 内转子速度
      | 的脉冲值
  Action Port : ActionPort
  Data Store Read1 : DataStoreRead  DataStoreName=Motor_Velocity  DataStoreElements=Motor_Velocity(5)
  Joint5_Velocity : Outport
  wires:
  Data Store Read1/1 -> Joint5_Velocity/1

== system PID_SingleJoint/DynamicsController/GetAngleVelocity/GetAngleSpeed2/Joint6 ==
  note: 内转子速度
      | 的脉冲值
  Action Port : ActionPort
  Data Store Read1 : DataStoreRead  DataStoreName=Motor_Velocity  DataStoreElements=Motor_Velocity(6)
  Joint6_Velocity : Outport
  wires:
  Data Store Read1/1 -> Joint6_Velocity/1

== system PID_SingleJoint/DynamicsController/GetAngleVelocity/GetAngleSpeed3/Joint1 ==
  note: 内转子速度
      | 的脉冲值
  Action Port : ActionPort
  Data Store Read1 : DataStoreRead  DataStoreName=Motor_Velocity  DataStoreElements=Motor_Velocity(1)
  Joint1_Velocity : Outport
  wires:
  Data Store Read1/1 -> Joint1_Velocity/1

== system PID_SingleJoint/DynamicsController/GetAngleVelocity/GetAngleSpeed3/Joint2 ==
  note: 内转子速度
      | 的脉冲值
  Action Port : ActionPort
  Data Store Read1 : DataStoreRead  DataStoreName=Motor_Velocity  DataStoreElements=Motor_Velocity(2)
  Joint2_Velocity : Outport
  wires:
  Data Store Read1/1 -> Joint2_Velocity/1

== system PID_SingleJoint/DynamicsController/GetAngleVelocity/GetAngleSpeed3/Joint3 ==
  note: 内转子速度
      | 的脉冲值
  Action Port : ActionPort
  Data Store Read1 : DataStoreRead  DataStoreName=Motor_Velocity  DataStoreElements=Motor_Velocity(3)
  Joint3_Velocity : Outport
  wires:
  Data Store Read1/1 -> Joint3_Velocity/1

== system PID_SingleJoint/DynamicsController/GetAngleVelocity/GetAngleSpeed3/Joint4 ==
  note: 内转子速度
      | 的脉冲值
  Action Port : ActionPort
  Data Store Read1 : DataStoreRead  DataStoreName=Motor_Velocity  DataStoreElements=Motor_Velocity(4)
  Joint4_Velocity : Outport
  wires:
  Data Store Read1/1 -> Joint4_Velocity/1

== system PID_SingleJoint/DynamicsController/GetAngleVelocity/GetAngleSpeed3/Joint5 ==
  note: 内转子速度
      | 的脉冲值
  Action Port : ActionPort
  Data Store Read1 : DataStoreRead  DataStoreName=Motor_Velocity  DataStoreElements=Motor_Velocity(5)
  Joint5_Velocity : Outport
  wires:
  Data Store Read1/1 -> Joint5_Velocity/1

== system PID_SingleJoint/DynamicsController/GetAngleVelocity/GetAngleSpeed3/Joint6 ==
  note: 内转子速度
      | 的脉冲值
  Action Port : ActionPort
  Data Store Read1 : DataStoreRead  DataStoreName=Motor_Velocity  DataStoreElements=Motor_Velocity(6)
  Joint6_Velocity : Outport
  wires:
  Data Store Read1/1 -> Joint6_Velocity/1

== system PID_SingleJoint/DynamicsController/GetAngleVelocity/GetAngleSpeed4/Joint1 ==
  note: 内转子速度
      | 的脉冲值
  Action Port : ActionPort
  Data Store Read1 : DataStoreRead  DataStoreName=Motor_Velocity  DataStoreElements=Motor_Velocity(1)
  Joint1_Velocity : Outport
  wires:
  Data Store Read1/1 -> Joint1_Velocity/1

== system PID_SingleJoint/DynamicsController/GetAngleVelocity/GetAngleSpeed4/Joint2 ==
  note: 内转子速度
      | 的脉冲值
  Action Port : ActionPort
  Data Store Read1 : DataStoreRead  DataStoreName=Motor_Velocity  DataStoreElements=Motor_Velocity(2)
  Joint2_Velocity : Outport
  wires:
  Data Store Read1/1 -> Joint2_Velocity/1

== system PID_SingleJoint/DynamicsController/GetAngleVelocity/GetAngleSpeed4/Joint3 ==
  note: 内转子速度
      | 的脉冲值
  Action Port : ActionPort
  Data Store Read1 : DataStoreRead  DataStoreName=Motor_Velocity  DataStoreElements=Motor_Velocity(3)
  Joint3_Velocity : Outport
  wires:
  Data Store Read1/1 -> Joint3_Velocity/1

== system PID_SingleJoint/DynamicsController/GetAngleVelocity/GetAngleSpeed4/Joint4 ==
  note: 内转子速度
      | 的脉冲值
  Action Port : ActionPort
  Data Store Read1 : DataStoreRead  DataStoreName=Motor_Velocity  DataStoreElements=Motor_Velocity(4)
  Joint4_Velocity : Outport
  wires:
  Data Store Read1/1 -> Joint4_Velocity/1

== system PID_SingleJoint/DynamicsController/GetAngleVelocity/GetAngleSpeed4/Joint5 ==
  note: 内转子速度
      | 的脉冲值
  Action Port : ActionPort
  Data Store Read1 : DataStoreRead  DataStoreName=Motor_Velocity  DataStoreElements=Motor_Velocity(5)
  Joint5_Velocity : Outport
  wires:
  Data Store Read1/1 -> Joint5_Velocity/1

== system PID_SingleJoint/DynamicsController/GetAngleVelocity/GetAngleSpeed4/Joint6 ==
  note: 内转子速度
      | 的脉冲值
  Action Port : ActionPort
  Data Store Read1 : DataStoreRead  DataStoreName=Motor_Velocity  DataStoreElements=Motor_Velocity(6)
  Joint6_Velocity : Outport
  wires:
  Data Store Read1/1 -> Joint6_Velocity/1

== system PID_SingleJoint/DynamicsController/GetAngleVelocity/GetAngleSpeed5/Joint1 ==
  note: 内转子速度
      | 的脉冲值
  Action Port : ActionPort
  Data Store Read1 : DataStoreRead  DataStoreName=Motor_Velocity  DataStoreElements=Motor_Velocity(1)
  Joint1_Velocity : Outport
  wires:
  Data Store Read1/1 -> Joint1_Velocity/1

== system PID_SingleJoint/DynamicsController/GetAngleVelocity/GetAngleSpeed5/Joint2 ==
  note: 内转子速度
      | 的脉冲值
  Action Port : ActionPort
  Data Store Read1 : DataStoreRead  DataStoreName=Motor_Velocity  DataStoreElements=Motor_Velocity(2)
  Joint2_Velocity : Outport
  wires:
  Data Store Read1/1 -> Joint2_Velocity/1

== system PID_SingleJoint/DynamicsController/GetAngleVelocity/GetAngleSpeed5/Joint3 ==
  note: 内转子速度
      | 的脉冲值
  Action Port : ActionPort
  Data Store Read1 : DataStoreRead  DataStoreName=Motor_Velocity  DataStoreElements=Motor_Velocity(3)
  Joint3_Velocity : Outport
  wires:
  Data Store Read1/1 -> Joint3_Velocity/1

== system PID_SingleJoint/DynamicsController/GetAngleVelocity/GetAngleSpeed5/Joint4 ==
  note: 内转子速度
      | 的脉冲值
  Action Port : ActionPort
  Data Store Read1 : DataStoreRead  DataStoreName=Motor_Velocity  DataStoreElements=Motor_Velocity(4)
  Joint4_Velocity : Outport
  wires:
  Data Store Read1/1 -> Joint4_Velocity/1

== system PID_SingleJoint/DynamicsController/GetAngleVelocity/GetAngleSpeed5/Joint5 ==
  note: 内转子速度
      | 的脉冲值
  Action Port : ActionPort
  Data Store Read1 : DataStoreRead  DataStoreName=Motor_Velocity  DataStoreElements=Motor_Velocity(5)
  Joint5_Velocity : Outport
  wires:
  Data Store Read1/1 -> Joint5_Velocity/1

== system PID_SingleJoint/DynamicsController/GetAngleVelocity/GetAngleSpeed5/Joint6 ==
  note: 内转子速度
      | 的脉冲值
  Action Port : ActionPort
  Data Store Read1 : DataStoreRead  DataStoreName=Motor_Velocity  DataStoreElements=Motor_Velocity(6)
  Joint6_Velocity : Outport
  wires:
  Data Store Read1/1 -> Joint6_Velocity/1

== system PID_SingleJoint/DynamicsController/DriveMotor/驱动器指令/Chart2/BG/J1_BG ==
  note: 命令
  note: 电流
  note: 位
      | 置
  Constant1 : Constant  Value=hex2dec('47')  OutDataTypeStr=uint8
  Constant2 : Constant  Value=0  VectorParams1D=off  OutDataTypeStr=uint8  SampleTime=-1
  Constant3 : Constant  Value=0  VectorParams1D=off  OutDataTypeStr=uint8  SampleTime=-1
  Constant8 : Constant  Value=hex2dec('42')  OutDataTypeStr=uint8
  Data Type Conversion : DataTypeConversion  OutDataTypeStr=uint16
  Data Type Conversion{1..6} (6 alike) : DataTypeConversion  OutDataTypeStr=uint8
  Mux3 : Mux  Inputs=8
  Shift Arithmetic1 : ArithShift  BitShiftNumber=8  BitShiftDirection=Right
  Shift Arithmetic2 : ArithShift  BitShiftNumber=16  BitShiftDirection=Right
  Shift Arithmetic3 : ArithShift  BitShiftNumber=24  BitShiftDirection=Right
  Shift Arithmetic4 : ArithShift  BitShiftNumber=8  BitShiftDirection=Right
  MSG : Outport
  wires:
  Shift Arithmetic2/1 -> Data Type Conversion4/1
  Shift Arithmetic4/1 -> Data Type Conversion6/1
  Constant2/1 -> Shift Arithmetic4/1, Data Type Conversion1/1
  Data Type Conversion1/1 -> Mux3/3
  Data Type Conversion3/1 -> Mux3/6
  Constant3/1 -> Data Type Conversion2/1, Shift Arithmetic1/1, Shift Arithmetic2/1, Shift Arithmetic3/1
  Data Type Conversion6/1 -> Mux3/4
  Shift Arithmetic3/1 -> Data Type Conversion5/1
  Shift Arithmetic1/1 -> Data Type Conversion3/1
  Mux3/1 -> Data Type Conversion/1
  Data Type Conversion2/1 -> Mux3/5
  Constant8/1 -> Mux3/1
  Data Type Conversion4/1 -> Mux3/7
  Data Type Conversion5/1 -> Mux3/8
  Constant1/1 -> Mux3/2
  Data Type Conversion/1 -> MSG/1

== system PID_SingleJoint/DynamicsController/DriveMotor/驱动器指令/Chart2/BG/J2_BG ==
  note: 位
      | 置
  note: 电流
  note: 命令
  Constant1 : Constant  Value=hex2dec('47')  OutDataTypeStr=uint8
  Constant2 : Constant  Value=0  VectorParams1D=off  OutDataTypeStr=uint8  SampleTime=-1
  Constant3 : Constant  Value=0  VectorParams1D=off  OutDataTypeStr=uint8  SampleTime=-1
  Constant8 : Constant  Value=hex2dec('42')  OutDataTypeStr=uint8
  Data Type Conversion : DataTypeConversion  OutDataTypeStr=uint16
  Data Type Conversion{1..6} (6 alike) : DataTypeConversion  OutDataTypeStr=uint8
  Mux3 : Mux  Inputs=8
  Shift Arithmetic1 : ArithShift  BitShiftNumber=8  BitShiftDirection=Right
  Shift Arithmetic2 : ArithShift  BitShiftNumber=16  BitShiftDirection=Right
  Shift Arithmetic3 : ArithShift  BitShiftNumber=24  BitShiftDirection=Right
  Shift Arithmetic4 : ArithShift  BitShiftNumber=8  BitShiftDirection=Right
  MSG : Outport
  wires:
  Data Type Conversion/1 -> MSG/1
  Constant1/1 -> Mux3/2
  Data Type Conversion5/1 -> Mux3/8
  Data Type Conversion4/1 -> Mux3/7
  Constant8/1 -> Mux3/1
  Data Type Conversion2/1 -> Mux3/5
  Mux3/1 -> Data Type Conversion/1
  Shift Arithmetic1/1 -> Data Type Conversion3/1
  Shift Arithmetic3/1 -> Data Type Conversion5/1
  Data Type Conversion6/1 -> Mux3/4
  Constant3/1 -> Shift Arithmetic3/1, Shift Arithmetic2/1, Shift Arithmetic1/1, Data Type Conversion2/1
  Data Type Conversion3/1 -> Mux3/6
  Data Type Conversion1/1 -> Mux3/3
  Constant2/1 -> Data Type Conversion1/1, Shift Arithmetic4/1
  Shift Arithmetic4/1 -> Data Type Conversion6/1
  Shift Arithmetic2/1 -> Data Type Conversion4/1
